simulink model "f14c"  (Simulink 6.0)
settings: Solver=ode23  SolverMode=SingleTasking  StartTime=0.0  StopTime=2  MaxStep=.01  RelTol=1e-4  AbsTol=1e-6
PreLoadFcn:
  | f14dat
values from neighbouring files (symbols this model uses):
  a = 2.5348    [autopilot_data.mat]    (also in f14dat.m; f14def.m)
  b = 64.13    [autopilot_data.mat]    (also in f14dat.m; f14def.m)
  Ka = 0.677    [autopilot_data.mat]    (also in f14dat.m; f14def.m)
  Kf = -1.746    [autopilot_data.mat]    (also in f14dat.m; f14def.m)
  Ki = -3.864    [autopilot_data.mat]    (also in f14dat.m; f14def.m)
  Kq = 0.8156    [autopilot_data.mat]    (also in f14dat.m; f14def.m)
  Md = -6.8847    [autopilot_data.mat]    (also in f14dat.m; f14def.m)
  Mq = -0.0164275    [autopilot_data.mat]    (also in f14dat.m = -0.6571; f14def.m = -0.6571)
  Mw = -0.000148    [autopilot_data.mat]    (also in f14dat.m = -0.00592; f14def.m = -0.00592)
  Sa = 0.005236    [autopilot_data.mat]    (also in f14dat.m; f14def.m)
  Swg = 3    [autopilot_data.mat]    (also in f14dat.m; f14def.m)
  Ta = 0.05    [autopilot_data.mat]    (also in f14dat.m; f14def.m)
  Tal = 0.3959    [autopilot_data.mat]    (also in f14dat.m; f14def.m)
  Ts = 0.2    [autopilot_data.mat]    (also in f14dat.m = 0.1; f14def.m = 0.1)
  Uo = 689.4    [autopilot_data.mat]    (also in f14dat.m; f14def.m)
  Vto = 690.4    [autopilot_data.mat]    (also in f14dat.m; f14def.m)
  W1 = 2.971    [autopilot_data.mat]    (also in f14dat.m; f14def.m)
  W2 = 4.144    [autopilot_data.mat]    (also in f14dat.m; f14def.m)
  Wa = 10    [autopilot_data.mat]    (also in f14dat.m; f14def.m)
  Zd = -63.9979    [autopilot_data.mat]    (also in f14dat.m; f14def.m)
  Zw = -0.0159625    [autopilot_data.mat]    (also in f14dat.m = -0.6385; f14def.m = -0.6385)
settings Model: Creator=The MathWorks Inc.  LastModifiedBy=batserve  ExtModeAutoUpdateStatusClock=off
settings DataIOCC: ExternalInput=[]  InitialState=[]  LimitDataPoints=off  SaveOutput=off  SaveTime=off
settings OptimizationCC: BooleanDataType=off
settings DebuggingCC: CheckExecutionContextPreStartOutputMsg=on  CheckExecutionContextRuntimeOutputMsg=on  SolverPrmCheckMsg=none
settings HardwareCC: TargetUnknown=on

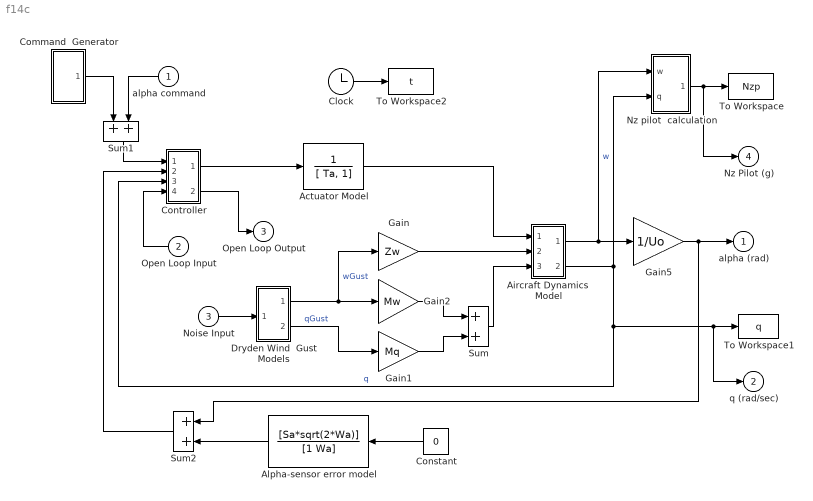
== system f14c ==
  alpha command : Inport  Orientation=left  Port=1  LatchInput=off
  Open Loop Input : Inport  Orientation=left  Port=2  LatchInput=off
  Noise Input : Inport  Port=3  LatchInput=off
  Actuator Model : TransferFcn  Denominator=[ Ta, 1]
  Aircraft Dynamics  Model : Subsystem  PropExecContextAcrossSSBoundary=on
  Alpha-sensor error model : TransferFcn  Orientation=left  Numerator=[Sa*sqrt(2*Wa)]  Denominator=[1 Wa]
  Clock : Clock
      settings: Decimation=10
  Command  Generator : Subsystem  PropExecContextAcrossSSBoundary=on
  Constant : Constant  Orientation=left  Value=0
  Controller : Subsystem  PropExecContextAcrossSSBoundary=on
  Dryden Wind  Gust Models : Subsystem  PropExecContextAcrossSSBoundary=on
  Gain : Gain  Gain=Zw  SaturateOnIntegerOverflow=on
  Gain1 : Gain  Gain=Mq  SaturateOnIntegerOverflow=on
  Gain2 : Gain  Gain=Mw  SaturateOnIntegerOverflow=on
  Gain5 : Gain  Gain=1/Uo  SaturateOnIntegerOverflow=on
  Nz pilot  calculation : Subsystem  PropExecContextAcrossSSBoundary=on
  Sum : Sum  SaturateOnIntegerOverflow=on  InputSameDT=on
  Sum1 : Sum  Orientation=down  SaturateOnIntegerOverflow=on  InputSameDT=on
  Sum2 : Sum  Orientation=left  SaturateOnIntegerOverflow=on  InputSameDT=on
  To Workspace : ToWorkspace  VariableName=Nzp  SampleTime=-1  SaveFormat=Array
  To Workspace1 : ToWorkspace  VariableName=q  SampleTime=-1  SaveFormat=Array
  To Workspace2 : ToWorkspace  VariableName=t  SampleTime=-1  SaveFormat=Array
  alpha (rad) : Outport  InitialOutput=0
  q (rad/sec) : Outport  Port=2  InitialOutput=0
  Open Loop Output : Outport  Port=3  InitialOutput=0
  Nz Pilot (g) : Outport  Port=4  InitialOutput=0
  wires:
  Clock/1 -> To Workspace2/1
  Command  Generator/1(alpha command) -> Sum1/1
  Controller/2(Open Loop Output) -> Open Loop Output/1
  Constant/1 -> Alpha-sensor error model/1
  Noise Input/1 -> Dryden Wind  Gust Models/1(Noise Input)
  Open Loop Input/1 -> Controller/4(Open Loop Input)
  Sum2/1 -> Controller/2(alpha (rad))
  Alpha-sensor error model/1 -> Sum2/2
  Sum1/1 -> Controller/1(Stick Input (in))
  Dryden Wind  Gust Models/1(wGust (ft/sec)) -> Gain2/1, Gain/1  "wGust"
  Controller/1(Elevator Command (deg)) -> Actuator Model/1
  Gain1/1 -> Sum/2
  Gain2/1 -> Sum/1
  Dryden Wind  Gust Models/2(qGust (rad/sec)) -> Gain1/1  "qGust"
  alpha command/1 -> Sum1/2
  Aircraft Dynamics  Model/2(Pitch Rate q (rad/sec)) -> Nz pilot  calculation/2(q), Controller/3(q (rad/sec)), To Workspace1/1, q (rad/sec)/1  "q"
  Aircraft Dynamics  Model/1(Vertical Velocity w (ft/sec)) -> Gain5/1, Nz pilot  calculation/1(w)  "w"
  Sum/1 -> Aircraft Dynamics  Model/3(Rotary Gust qGust (rad/sec))
  Gain/1 -> Aircraft Dynamics  Model/2(Vertical Gust wGust (ft/sec))
  Actuator Model/1 -> Aircraft Dynamics  Model/1(Elevator Deflection d (deg))
  Nz pilot  calculation/1(Pilot g force (g)) -> To Workspace/1, Nz Pilot (g)/1
  Gain5/1 -> alpha (rad)/1, Sum2/1

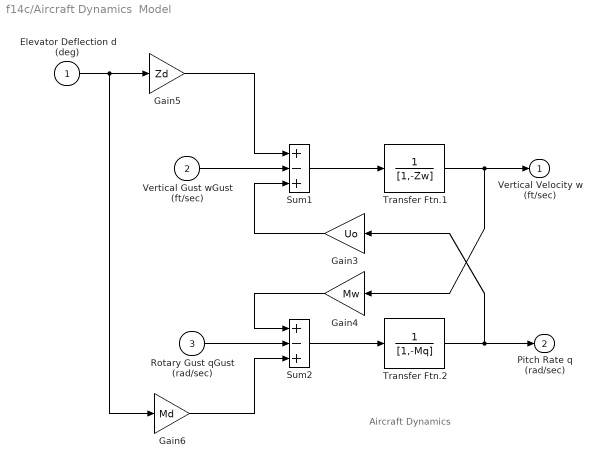
== system f14c/Aircraft Dynamics  Model ==
  note: Aircraft Dynamics
  Elevator Deflection d (deg) : Inport  Port=1  LatchInput=off
  Vertical Gust wGust (ft/sec) : Inport  Port=2  LatchInput=off
  Rotary Gust qGust (rad/sec) : Inport  Port=3  LatchInput=off
  Gain3 : Gain  Orientation=left  Gain=Uo  SaturateOnIntegerOverflow=on
  Gain4 : Gain  Orientation=left  Gain=Mw  SaturateOnIntegerOverflow=on
  Gain5 : Gain  Gain=Zd  SaturateOnIntegerOverflow=on
  Gain6 : Gain  Gain=Md  SaturateOnIntegerOverflow=on
  Sum1 : Sum  Inputs=+-+  SaturateOnIntegerOverflow=on  InputSameDT=on
  Sum2 : Sum  Inputs=+-+  SaturateOnIntegerOverflow=on  InputSameDT=on
  "Transfer Ftn.1 " : TransferFcn  Denominator=[1,-Zw]
  Transfer Ftn.2 : TransferFcn  Denominator=[1,-Mq]
  Vertical Velocity w (ft/sec) : Outport  InitialOutput=0
  Pitch Rate q (rad/sec) : Outport  Port=2  InitialOutput=0
  wires:
  "Transfer Ftn.1 "/1 -> Vertical Velocity w (ft/sec)/1, Gain4/1
  Transfer Ftn.2/1 -> Pitch Rate q (rad/sec)/1, Gain3/1
  Gain6/1 -> Sum2/3
  Gain5/1 -> Sum1/1
  Gain3/1 -> Sum1/3
  Rotary Gust qGust (rad/sec)/1 -> Sum2/2
  Sum2/1 -> Transfer Ftn.2/1
  Sum1/1 -> "Transfer Ftn.1 "/1
  Gain4/1 -> Sum2/1
  Vertical Gust wGust (ft/sec)/1 -> Sum1/2
  Elevator Deflection d (deg)/1 -> Gain5/1, Gain6/1

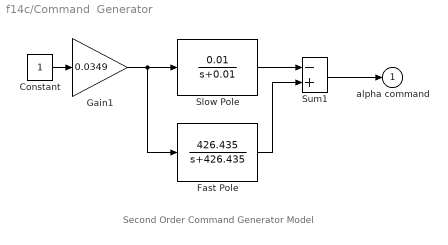
== system f14c/Command  Generator ==
  note: Second Order Command Generator Model
  Constant : Constant
  Fast Pole : TransferFcn  Numerator=[426.435]  Denominator=[ 1 426.435]
  Gain1 : Gain  Gain=0.0349  SaturateOnIntegerOverflow=on
  Slow Pole : TransferFcn  Numerator=[0.01]  Denominator=[ 1 0.01]
  Sum1 : Sum  Inputs=-+  SaturateOnIntegerOverflow=on  InputSameDT=on
  alpha command : Outport  InitialOutput=0
  wires:
  Gain1/1 -> Slow Pole/1, Fast Pole/1
  Constant/1 -> Gain1/1
  Fast Pole/1 -> Sum1/2
  Slow Pole/1 -> Sum1/1
  Sum1/1 -> alpha command/1

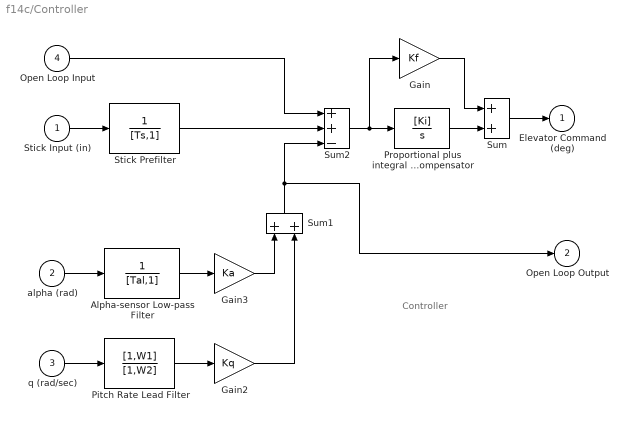
== system f14c/Controller ==
  note: Controller
  Stick Input (in) : Inport  Port=1  LatchInput=off
  alpha (rad) : Inport  Port=2  LatchInput=off
  q (rad/sec) : Inport  Port=3  LatchInput=off
  Open Loop Input : Inport  Port=4  LatchInput=off
  Alpha-sensor Low-pass Filter : TransferFcn  Denominator=[Tal,1]
  Gain : Gain  Gain=Kf  SaturateOnIntegerOverflow=on
  Gain2 : Gain  Gain=Kq  SaturateOnIntegerOverflow=on
  Gain3 : Gain  Gain=Ka  SaturateOnIntegerOverflow=on
  Pitch Rate Lead Filter : TransferFcn  Numerator=[1,W1]  Denominator=[1,W2]
  Proportional plus integral compensator : TransferFcn  Numerator=[Ki]  Denominator=[1,0]
  Stick Prefilter : TransferFcn  Denominator=[Ts,1]
  Sum : Sum  Inputs=2  SaturateOnIntegerOverflow=on  InputSameDT=on
  Sum1 : Sum  Orientation=up  Inputs=2  SaturateOnIntegerOverflow=on  InputSameDT=on
  Sum2 : Sum  Inputs=++-  SaturateOnIntegerOverflow=on  InputSameDT=on
  Elevator Command (deg) : Outport  InitialOutput=0
  Open Loop Output : Outport  Port=2  InitialOutput=0
  wires:
  Sum1/1 -> Open Loop Output/1, Sum2/3
  Sum2/1 -> Proportional plus integral compensator/1, Gain/1
  Gain/1 -> Sum/1
  Proportional plus integral compensator/1 -> Sum/2
  Stick Input (in)/1 -> Stick Prefilter/1
  Sum/1 -> Elevator Command (deg)/1
  Pitch Rate Lead Filter/1 -> Gain2/1
  q (rad/sec)/1 -> Pitch Rate Lead Filter/1
  Alpha-sensor Low-pass Filter/1 -> Gain3/1
  alpha (rad)/1 -> Alpha-sensor Low-pass Filter/1
  Gain3/1 -> Sum1/1
  Gain2/1 -> Sum1/2
  Stick Prefilter/1 -> Sum2/2
  Open Loop Input/1 -> Sum2/1

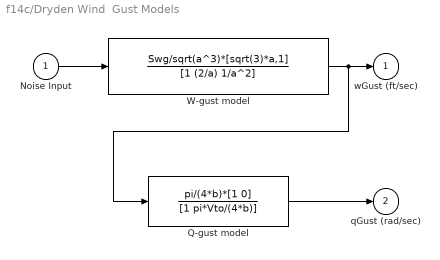
== system f14c/Dryden Wind  Gust Models ==
  Noise Input : Inport  Port=1  LatchInput=off
  Q-gust model : TransferFcn  Numerator=pi/(4*b)*[1 0]  Denominator=[1 pi*Vto/(4*b)]
  W-gust model : TransferFcn  Numerator=Swg/sqrt(a^3)*[sqrt(3)*a,1]  Denominator=[1 (2/a) 1/a^2]
  wGust (ft/sec) : Outport  InitialOutput=0
  qGust (rad/sec) : Outport  Port=2  InitialOutput=0
  wires:
  Noise Input/1 -> W-gust model/1
  Q-gust model/1 -> qGust (rad/sec)/1
  W-gust model/1 -> wGust (ft/sec)/1, Q-gust model/1

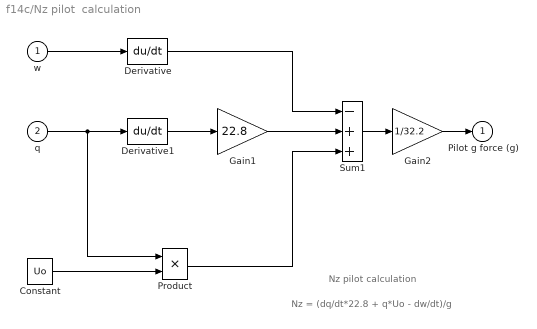
== system f14c/Nz pilot  calculation ==
  note: Nz = (dq/dt*22.8 + q*Uo - dw/dt)/g
  note: Nz pilot calculation
  w : Inport  Port=1  LatchInput=off
  q : Inport  Port=2  LatchInput=off
  Constant : Constant  Value=Uo
  Derivative : Derivative
  Derivative1 : Derivative
  Gain1 : Gain  Gain=22.8  SaturateOnIntegerOverflow=on
  Gain2 : Gain  Gain=1/32.2  SaturateOnIntegerOverflow=on
  Product : Product  SaturateOnIntegerOverflow=on  RndMeth=Zero  InputSameDT=on
  Sum1 : Sum  Inputs=-++  SaturateOnIntegerOverflow=on  InputSameDT=on
  Pilot g force (g) : Outport  InitialOutput=0
  wires:
  q/1 -> Product/1, Derivative1/1
  Constant/1 -> Product/2
  Gain2/1 -> Pilot g force (g)/1
  Sum1/1 -> Gain2/1
  Derivative/1 -> Sum1/1
  w/1 -> Derivative/1
  Derivative1/1 -> Gain1/1
  Gain1/1 -> Sum1/2
  Product/1 -> Sum1/3
